simulink library "sm_trackV_lib_chain_underc_i2u0l4"  (R2026a)
settings: Solver=VariableStepAuto
undefined symbols (not defined in the file): Excv, P1, P2, P3, P4, Right
libraries: sm_trackV_lib_chain_underc_elem x9, sm_lib x8, nesl_utility x7, fl_lib x2, sm_trackV_lib_frame_i2u0l4 x1
Description:
  | Copyright 2023-2026 The MathWorks, Inc.
settings Model: Creator=smiller  LastModifiedBy=smiller

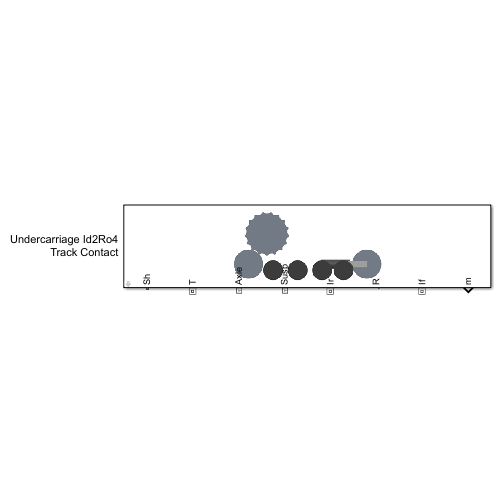
[thumbnail: Simulink's stored preview of the top-level diagram]
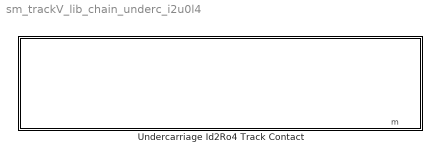
== system sm_trackV_lib_chain_underc_i2u0l4 ==
  Undercarriage Id2Ro4 Track Contact : Subsystem  mask(Undercarriage for Integration with Track Model){popup_leftOrRight=Right, sprk_xc=Excv.Sprocket.sprocket_xc, sprk_len=Excv.Sprocket.sprk_width, sprk_rho=Excv.Sprocket.density, sprk_clr=Excv.Sprocket.clr, sprk_opc=Excv.Sprocket.opc, sprk_contact_geo_ptcld=Excv.Sprocket.teeth_contact.ptcld.pts, sprk_contact_geo_rad=Excv.Sprocket.teeth_contact.ptcld.rad, sprk_contact_geo_clr=Excv.Sprocket.teeth_contact.ptcld.clr, sprk_contact_geo_opc=Excv.Sprocket.teeth_contact.ptcld.opc, idlerR_rad=Excv.IdlerR.rad, idlerF_rad=Excv.IdlerF.rad, idlerR_len=Excv.IdlerR.len, idlerF_len=Excv.IdlerF.len, idlerR_rho=Excv.IdlerR.rho, idlerF_rho=Excv.IdlerF.rho, idlerR_clr=Excv.IdlerR.clr, idlerF_clr=Excv.IdlerF.clr, idlerR_opc=Excv.IdlerR.opc, idlerF_opc=Excv.IdlerF.opc, idlerR_contgeo_clr=Excv.IdlerR.chain_contact.clr, idlerF_contgeo_clr=Excv.IdlerF.chain_contact.clr, idlerR_contgeo_opc=Excv.IdlerR.chain_contact.opc, idlerF_contgeo_opc=Excv.IdlerF.chain_contact.opc, roller_lower_rad=Excv.Roller.Lower.rad, roller_lower_len=Excv.Roller.Lower.len, roller_lower_rho=Excv.Roller.Lower.rho, roller_lower_clr=Excv.Roller.Lower.clr, roller_lower_opc=Excv.Roller.Lower.opc, roller_lower_contgeo_clr=[1.0 0.0 0.0], roller_lower_contgeo_opc=1, tensioner_cyl_len=Excv.IdlerF.Tensioner.cyl.len, tensioner_cyl_rad=Excv.IdlerF.Tensioner.cyl.rad, tensioner_cyl_rho=Excv.IdlerF.Tensioner.cyl.rho, tensioner_cyl_clr=Excv.IdlerF.Tensioner.cyl.clr, tensioner_cyl_opc=Excv.IdlerF.Tensioner.cyl.opc, tensioner_pist_len=Excv.IdlerF.Tensioner.piston.len, tensioner_pist_rad=Excv.IdlerF.Tensioner.piston.rad, tensioner_pist_rho=Excv.IdlerF.Tensioner.piston.rho, tensioner_pist_clr=Excv.IdlerF.Tensioner.piston.clr, tensioner_pist_opc=Excv.IdlerF.Tensioner.piston.opc, tensioner_br_len=Excv.IdlerF.Tensioner.bracket.len, tensioner_br_width=Excv.IdlerF.Tensioner.bracket.wid, tensioner_br_height=Excv.IdlerF.Tensioner.bracket.height, tensioner_br_thk=Excv.IdlerF.Tensioner.bracket.thk, tensioner_br_rho=Excv.IdlerF.Tensioner.bracket.rho, tensioner_br_clr=Excv.IdlerF.Tensioner.bracket.clr, tensioner_br_opc=Excv.IdlerF.Tensioner.bracket.opc, tensioner_eqpos=Excv.IdlerF.Tensioner.xeq, tensioner_x0=Excv.IdlerF.Tensioner.x0, tensioner_k=Excv.IdlerF.Tensioner.K, tensioner_b=Excv.IdlerF.Tensioner.B, roller_lower_x=Excv.Frame.Sprk2LowerX, idlerF_x=Excv.Frame.IdlerAssyX, idlerR_x=Excv.Frame.Sprk2IdlerRX, axle_x=Excv.Frame.AxleX, roller_lower_y=Excv.Frame.Sprk2LowerY, idlerF_y=Excv.Frame.Sprk2IdlerFY, idlerR_y=Excv.Frame.Sprk2IdlerFY, axle_y=Excv.Frame.AxleY, frame_cg_offset=Excv.Frame.CGOffset, frame_mass=Excv.Frame.Mass, frame_moi=Excv.Frame.MOI, frame_poi=Excv.Frame.POI, frame_susp_offset=Excv.Frame.SuspOffset, popup_sense_roller=Actuator Torque}
      mask prompts: popup_leftOrRight "Left or Right"; sprk_xc "Extrusion Data [x y] (m)"; sprk_len "Length (m)"; sprk_rho "Density (kg/m^3)"; sprk_clr "Color [R G B] (0-1)"; sprk_opc "Opacity (0-1)"; sprk_contact_geo_ptcld "Point Cloud Data [x y z] (m)"; sprk_contact_geo_rad "Radius (m)"; sprk_contact_geo_clr "Color [R G B] (0-1)"; sprk_contact_geo_opc "Opacity (0-1)"; roller_lower_rad "Radius (m)"; roller_lower_len "Length (m)"; roller_lower_rho "Density (kg/m^3)"; roller_lower_clr "Color [R G B] (0-1)"; roller_lower_opc "Opacity (0-1)"; roller_lower_contgeo_clr "Color [R G B] (0-1)"; roller_lower_contgeo_opc "Opacity (0-1)"; tensioner_cyl_len "Length (m)"; tensioner_cyl_rad "Radius (m)"; tensioner_cyl_rho "Density (kg/m^3)"; tensioner_cyl_clr "Color [R G B] (0-1)"; tensioner_cyl_opc "Opacity (0-1)"; tensioner_pist_len "Piston Length (m)"; tensioner_pist_rad "Radius (m)"; tensioner_pist_rho "Density (kg/m^3)"; tensioner_pist_clr "Color [R G B] (0-1)"; tensioner_pist_opc "Opacity (0.1)"; tensioner_br_len "Length (m)"; tensioner_br_width "Width (m)"; tensioner_br_height "Height (m)"; tensioner_br_thk "Bracket Thickness (m)"; tensioner_br_rho "Density (kg/m^3)"; tensioner_br_clr "Color [R G B] (0-1)"; tensioner_br_opc "Opacity (0.1)"; tensioner_eqpos "Equilibrium Position (m)"; tensioner_x0 "Assembly Position (m)"; tensioner_k "Stiffness Coefficient (N/m)"; tensioner_b "Damping Coefficient (N/(m/s))"; roller_lower_x "Lower Rollers (vector) (m)"; idlerF_x "Idler Wheel Front (m)"; idlerR_x "Idler Wheel Rear (m)"; axle_x "Axle (m)"; roller_lower_y "Lower Rollers (m)"; idlerF_y "Idler Front (m)"; idlerR_y "Idler Rear (m)"; axle_y "Axle (m)"; frame_cg_offset "CG Offset from Sprocket [x y z] (m)"; frame_mass "Mass (kg)"; frame_moi "Moments of Inertia [Ixx Iyy Izz] (kg*m^2)"; frame_poi "Products of Inertia [Ixx Iyy Izz] (kg*m^2)"; frame_susp_offset "Suspension Offset from Sprocket [x y z] (m)"; popup_sense_roller "Roller"
      mask help: Models sprocket, rollers, and idler with tensioner. Components have contact geometry for integration with a segmented track model. The sprocket has a 1D rotational mechanical interface to the drivetrain.
      mask init:
      | bh = gcb;
      | set_param([bh '/Rollers'],'popup_sense_roller',get_param(bh,'popup_sense_roller'));
      mask TypeOptions popup_leftOrRight: Frame/popup_leftOrRight
      mask TypeOptions sprk_xc: Rollers/sprk_xc
      mask TypeOptions sprk_len: Rollers/sprk_len
      mask TypeOptions sprk_rho: Rollers/sprk_rho
      mask TypeOptions sprk_clr: Rollers/sprk_clr
      mask TypeOptions sprk_opc: Rollers/sprk_opc
      mask TypeOptions sprk_contact_geo_ptcld: Rollers/sprk_contact_geo_ptcld
      mask TypeOptions sprk_contact_geo_rad: Rollers/sprk_contact_geo_rad
      mask TypeOptions sprk_contact_geo_clr: Rollers/sprk_contact_geo_clr
      mask TypeOptions sprk_contact_geo_opc: Rollers/sprk_contact_geo_opc
      mask TypeOptions idlerR_rad: Rollers/idlerR_rad
      mask TypeOptions idlerF_rad: Rollers/idlerF_rad
      mask TypeOptions idlerR_len: Rollers/idlerR_len
      mask TypeOptions idlerF_len: Rollers/idlerF_len
      mask TypeOptions idlerR_rho: Rollers/idlerR_rho
      mask TypeOptions idlerF_rho: Rollers/idlerF_rho
      mask TypeOptions idlerR_clr: Rollers/idlerR_clr
      mask TypeOptions idlerF_clr: Rollers/idlerF_clr
      mask TypeOptions idlerR_opc: Rollers/idlerR_opc
      mask TypeOptions idlerF_opc: Rollers/idlerF_opc
      mask TypeOptions idlerR_contgeo_clr: Rollers/idlerR_contgeo_clr
      mask TypeOptions idlerF_contgeo_clr: Rollers/idlerF_contgeo_clr
      mask TypeOptions idlerR_contgeo_opc: Rollers/idlerR_contgeo_opc
      mask TypeOptions idlerF_contgeo_opc: Rollers/idlerF_contgeo_opc
      mask TypeOptions roller_lower_rad: Rollers/roller_lower_rad
      mask TypeOptions roller_lower_len: Rollers/roller_lower_len
      mask TypeOptions roller_lower_rho: Rollers/roller_lower_rho
      mask TypeOptions roller_lower_clr: Rollers/roller_lower_clr
      mask TypeOptions roller_lower_opc: Rollers/roller_lower_opc
      mask TypeOptions roller_lower_contgeo_clr: Rollers/roller_lower_contgeo_clr
      mask TypeOptions roller_lower_contgeo_opc: Rollers/roller_lower_contgeo_opc
      mask TypeOptions tensioner_cyl_len: Rollers/tensioner_cyl_len
      mask TypeOptions tensioner_cyl_rad: Rollers/tensioner_cyl_rad
      mask TypeOptions tensioner_cyl_rho: Rollers/tensioner_cyl_rho
      mask TypeOptions tensioner_cyl_clr: Rollers/tensioner_cyl_clr
      mask TypeOptions tensioner_cyl_opc: Rollers/tensioner_cyl_opc
      mask TypeOptions tensioner_pist_len: Rollers/pist_len
      mask TypeOptions tensioner_pist_rad: Rollers/tensioner_pist_rad
      mask TypeOptions tensioner_pist_rho: Rollers/tensioner_pist_rho
      mask TypeOptions tensioner_pist_clr: Rollers/tensioner_pist_clr
      mask TypeOptions tensioner_pist_opc: Rollers/tensioner_pist_opc
      mask TypeOptions tensioner_br_len: Rollers/brk_len
      mask TypeOptions tensioner_br_width: Rollers/tensioner_br_width
      mask TypeOptions tensioner_br_height: Rollers/tensioner_br_height
      mask TypeOptions tensioner_br_thk: Rollers/brk_thk
      mask TypeOptions tensioner_br_rho: Rollers/tensioner_br_rho
      mask TypeOptions tensioner_br_clr: Rollers/tensioner_br_clr
      mask TypeOptions tensioner_br_opc: Rollers/tensioner_br_opc
      mask TypeOptions tensioner_eqpos: Rollers/tensioner_eqpos
      mask TypeOptions tensioner_x0: Rollers/tensioner_x0
      mask TypeOptions tensioner_k: Rollers/tensioner_k
      mask TypeOptions tensioner_b: Rollers/tensioner_b
      mask TypeOptions roller_lower_x: Frame/roller_lower_x
      mask TypeOptions idlerF_x: Frame/idlerF_x
      mask TypeOptions idlerR_x: Frame/idlerR_x
      mask TypeOptions axle_x: Frame/axle_x
      mask TypeOptions roller_lower_y: Frame/roller_lower_y
      mask TypeOptions idlerF_y: Frame/idlerF_y
      mask TypeOptions idlerR_y: Frame/idlerR_y
      mask TypeOptions axle_y: Frame/axle_y
      mask TypeOptions frame_cg_offset: Frame/frame_cg_offset
      mask TypeOptions frame_mass: Frame/frame_mass
      mask TypeOptions frame_moi: Frame/frame_moi
      mask TypeOptions frame_poi: Frame/frame_poi
      mask TypeOptions frame_susp_offset: Frame/frame_susp_offset
      mask TypeOptions popup_sense_roller: Constraint Force | Actuator Torque
      mask DialogControl cont_sprocket Prompt: Sprocket
      mask DialogControl cont_sprocket_solid Prompt: Solid
      mask DialogControl cont_sprocket_contact_geo Prompt: Contact Geometry
      mask DialogControl cont_idler Prompt: Idler
      mask DialogControl cont_idler_solid Prompt: Solid
      mask DialogControl text_rear Prompt: Rear
      mask DialogControl text_front Prompt: Front
      mask DialogControl text_rad Prompt: Radius (m)
      mask DialogControl text_len Prompt: Length (m)
      mask DialogControl text_rho Prompt: Density (kg/m^3)
      mask DialogControl text_clr Prompt: Color [R G B] (0-1)
      mask DialogControl text_opc Prompt: Opacity (0-1)
      mask DialogControl cont_idler_contact_geo Prompt: Contact Geometry
      mask DialogControl text_contgeo_clr Prompt: Color [R G B] (0-1)
      mask DialogControl text_contgeo_opc Prompt: Opacity (0-1)
      mask DialogControl cont_rollers Prompt: Rollers
      mask DialogControl cont_rollers_lower Prompt: Lower
      mask DialogControl cont_rollers_lower_contact_geo Prompt: Contact Geometry
      mask DialogControl cont_tensioner Prompt: Tensioner
      mask DialogControl cont_tensioner_cyl Prompt: Cylinder
      mask DialogControl cont_tensioner_pist Prompt: Piston
      mask DialogControl cont_tensioner_brkt Prompt: Bracket
      mask DialogControl cont_tensioner_assembly Prompt: Assembly
      mask DialogControl cont_frame Prompt: Frame
      mask DialogControl cont_offset_x Prompt: Longitudinal Offsets from Sprocket
      mask DialogControl cont_offset_y Prompt: Vertical Offsets
      mask DialogControl cont_mass Prompt: Mass and Inertia
      mask DialogControl cont_susp Prompt: Suspension Offsets
      mask DialogControl cont_sensing Prompt: Sensing
      mask Display: image('sm_chain_underc_i2u0l4_IMAGE.png');

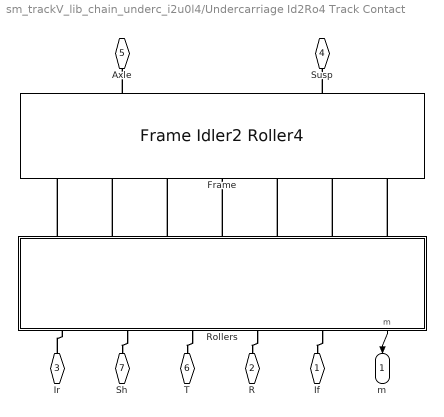
== system sm_trackV_lib_chain_underc_i2u0l4/Undercarriage Id2Ro4 Track Contact ==
  Frame : sm_trackV_lib_frame_i2u0l4/Frame Idler2 Roller4  popup_leftOrRight=Right  roller_lower_x=roller_lower_x  idlerF_x=idlerF_x  idlerR_x=idlerR_x  axle_x=axle_x  roller_lower_y=roller_lower_y  idlerF_y=idlerF_y  idlerR_y=idlerR_y  axle_y=axle_y  frame_cg_offset=frame_cg_offset  frame_mass=frame_mass  frame_moi=frame_moi  frame_poi=frame_poi  frame_susp_offset=frame_susp_offset
  Rollers : Subsystem  mask(Rollers for Integration with Track Model){sprk_xc=sprk_xc, sprk_len=sprk_len, sprk_rho=sprk_rho, sprk_clr=sprk_clr, sprk_opc=sprk_opc, sprk_contact_geo_ptcld=sprk_contact_geo_ptcld, sprk_contact_geo_rad=sprk_contact_geo_rad, sprk_contact_geo_clr=sprk_contact_geo_clr, sprk_contact_geo_opc=sprk_contact_geo_opc, idlerR_rad=idlerR_rad, idlerF_rad=idlerF_rad, idlerR_len=idlerR_len, idlerF_len=idlerF_len, idlerR_rho=idlerR_rho, idlerF_rho=idlerF_rho, idlerR_clr=idlerR_clr, idlerF_clr=idlerF_clr, idlerR_opc=idlerR_opc, idlerF_opc=idlerF_opc, idlerR_contgeo_clr=idlerR_contgeo_clr, idlerF_contgeo_clr=idlerF_contgeo_clr, idlerR_contgeo_opc=idlerR_contgeo_opc, idlerF_contgeo_opc=idlerF_contgeo_opc, roller_lower_len=roller_lower_len, roller_lower_rad=roller_lower_rad, roller_lower_rho=roller_lower_rho, roller_lower_clr=roller_lower_clr, roller_lower_opc=roller_lower_opc, roller_lower_contgeo_clr=roller_lower_contgeo_clr, roller_lower_contgeo_opc=roller_lower_contgeo_opc, tensioner_cyl_rad=tensioner_cyl_rad, tensioner_cyl_len=tensioner_cyl_len, tensioner_cyl_rho=tensioner_cyl_rho, tensioner_cyl_clr=tensioner_cyl_clr, tensioner_cyl_opc=tensioner_cyl_opc, tensioner_pist_rad=tensioner_pist_rad, pist_len=tensioner_pist_len, tensioner_pist_rho=tensioner_pist_rho, tensioner_pist_clr=tensioner_pist_clr, tensioner_pist_opc=tensioner_pist_opc, brk_len=tensioner_br_len, tensioner_br_width=tensioner_br_width, tensioner_br_height=tensioner_br_height, brk_thk=tensioner_br_thk, tensioner_br_rho=tensioner_br_rho, tensioner_br_clr=tensioner_br_clr, tensioner_br_opc=tensioner_br_opc, tensioner_eqpos=tensioner_eqpos, tensioner_x0=tensioner_x0, tensioner_b=tensioner_b, tensioner_k=tensioner_k, popup_sense_roller=Actuator Torque}
      mask prompts: sprk_xc "Extrusion Data [x y] (m)"; sprk_len "Length (m)"; sprk_rho "Density (kg/m^3)"; sprk_clr "Color [R G B] (0-1)"; sprk_opc "Opacity (0-1)"; sprk_contact_geo_ptcld "Point Cloud Data [x y z] (m)"; sprk_contact_geo_rad "Radius (m)"; sprk_contact_geo_clr "Color [R G B] (0-1)"; sprk_contact_geo_opc "Opacity (0-1)"; roller_lower_len "Length (m)"; roller_lower_rad "Radius (m)"; roller_lower_rho "Density (kg/m^3)"; roller_lower_clr "Color [R G B] (0-1)"; roller_lower_opc "Opacity (0-1)"; roller_lower_contgeo_clr "Color [R G B] (0-1)"; roller_lower_contgeo_opc "Opacity (0-1)"; tensioner_cyl_rad "Radius (m)"; tensioner_cyl_len "Length (m)"; tensioner_cyl_rho "Density (kg/m^3)"; tensioner_cyl_clr "Color [R G B] (0-1)"; tensioner_cyl_opc "Opacity (0-1)"; tensioner_pist_rad "Radius (m)"; pist_len "Piston Length (m)"; tensioner_pist_rho "Density (kg/m^3)"; tensioner_pist_clr "Color [R G B] (0-1)"; tensioner_pist_opc "Opacity (0.1)"; brk_len "Bracket Length (m)"; tensioner_br_width "Width (m)"; tensioner_br_height "Height (m)"; brk_thk "Bracket Thickness (m)"; tensioner_br_rho "Density (kg/m^3)"; tensioner_br_clr "Color [R G B] (0-1)"; tensioner_br_opc "Opacity (0.1)"; tensioner_eqpos "Equilibrium Position (m)"; tensioner_x0 "Assembly Position (m)"; tensioner_b "Damping Coefficient (N/(m/s))"; tensioner_k "Stiffness Coefficient (N/m)"; popup_sense_roller "Roller"
      mask help: Models sprocket, rollers, and idler with tensioner. Components have contact geometry for integration with a segmented track model. The sprocket has a 1D rotational mechanical interface to the drivetrain.
      mask init:
      | % Sensing a constraint force can be computationally expensive
      | % Use popup to turn it off if quantity is not needed
      | bh = gcb;
      | if(strcmp(get_param(bh,'popup_sense_roller'),'Constraint Force'))
      |     SCF = 'on'; STF = 'off';
      |     connectedPort = "fc_out";
      |     senseConstraintTorque = "on";
      |     senseTorqueForce = "off";
      | else
      |     SCF = 'off'; STF = 'on';
      |     connectedPort = "t_out";
      |     senseConstraintTorque = "off";
      |     senseTorqueForce = "on";
      | end
      | f = Simulink.FindOptions('RegExp',true,'SearchDepth',1);
      | bh_rv = Simulink.findBlocks(bh,'Name','Revolute Lower #*',f);
      | bh_ps = Simulink.findBlocks(bh,'Name','PS-SL Lower #*',f);
      | [~, indrv] = sort(getfullname(bh_rv));
      | [~, indps] = sort(getfullname(bh_ps));
      | bh_rv = bh_rv(indrv);
      | bh_ps = bh_ps(indps);
      | 
      | bh_rvidf = get_param([bh '/Revolute Idler F'],'Handle');
      | bh_rvidr = get_param([bh '/Revolute Idler R'],'Handle');
      | 
      | bh_psidf = get_param([bh '/PS-SL IdlerF'],'Handle');
      | bh_psidr = get_param([bh '/PS-SL IdlerR'],'Handle');
      | 
      | bh_rv = [bh_rv; bh_rvidr; bh_rvidf];
      | bh_ps = [bh_ps; bh_psidr; bh_psidf];
      | 
      | for i = 1:length(bh_rv)
      |     port_rv = get_param(bh_rv(i),'PortHandles');
      |     port_ps = get_param(bh_ps(i),'PortHandles');
      |     line_rv = get_param(bh_rv(i),'LineHandles');
      |     delete_line(line_rv.RConn(2))
      |     set_param(bh_rv(i),'SenseConstraintForce',SCF,'SenseTorqueForce',STF);
      |     %port_rv = get_param(bh_rv(1),'PortHandles')
      |     %add_line(bh,port_rv.RConn(2),port_ps.LConn,'autorouting','on');
      |     simscape.addConnection(bh_rv(i), connectedPort, bh_ps(i),'input');
      | end
      mask TypeOptions sprk_xc: Sprocket/sprk_xc
      mask TypeOptions sprk_len: Sprocket/sprk_len
      mask TypeOptions sprk_rho: Sprocket/sprk_rho
      mask TypeOptions sprk_clr: Sprocket/sprk_clr
      mask TypeOptions sprk_opc: Sprocket/sprk_opc
      mask TypeOptions sprk_contact_geo_ptcld: Sprocket/sprk_contact_geo_ptcld
      mask TypeOptions sprk_contact_geo_rad: Sprocket/sprk_contact_geo_rad
      mask TypeOptions sprk_contact_geo_clr: Sprocket/sprk_contact_geo_clr
      mask TypeOptions sprk_contact_geo_opc: Sprocket/sprk_contact_geo_opc
      mask TypeOptions idlerR_rad: IdlerR/idler_rad
      mask TypeOptions idlerF_rad: IdlerF/idler_rad
      mask TypeOptions idlerR_len: IdlerR/idler_len
      mask TypeOptions idlerF_len: IdlerF/idler_len
      mask TypeOptions idlerR_rho: IdlerR/idler_rho
      mask TypeOptions idlerF_rho: IdlerF/idler_rho
      mask TypeOptions idlerR_clr: IdlerR/idler_clr
      mask TypeOptions idlerF_clr: IdlerF/idler_clr
      mask TypeOptions idlerR_opc: IdlerR/idler_opc
      mask TypeOptions idlerF_opc: IdlerF/idler_opc
      mask TypeOptions idlerR_contgeo_clr: IdlerR/idler_contgeo_clr
      mask TypeOptions idlerF_contgeo_clr: IdlerF/idler_contgeo_clr
      mask TypeOptions idlerR_contgeo_opc: IdlerR/idler_contgeo_opc
      mask TypeOptions idlerF_contgeo_opc: IdlerF/idler_contgeo_opc
      mask TypeOptions roller_lower_len:
      | Roller
      | Lower 1/roller_lower_len | Roller
      | Lower 2/roller_lower_len | Roller
      | Lower 3/roller_lower_len | Roller
      | Lower 4/roller_lower_len
      mask TypeOptions roller_lower_rad:
      | Roller
      | Lower 1/roller_lower_rad | Roller
      | Lower 2/roller_lower_rad | Roller
      | Lower 3/roller_lower_rad | Roller
      | Lower 4/roller_lower_rad
      mask TypeOptions roller_lower_rho:
      | Roller
      | Lower 1/roller_lower_rho | Roller
      | Lower 2/roller_lower_rho | Roller
      | Lower 3/roller_lower_rho | Roller
      | Lower 4/roller_lower_rho
      mask TypeOptions roller_lower_clr:
      | Roller
      | Lower 1/roller_lower_clr | Roller
      | Lower 2/roller_lower_clr | Roller
      | Lower 3/roller_lower_clr | Roller
      | Lower 4/roller_lower_clr
      mask TypeOptions roller_lower_opc:
      | Roller
      | Lower 1/roller_lower_opc | Roller
      | Lower 2/roller_lower_opc | Roller
      | Lower 3/roller_lower_opc | Roller
      | Lower 4/roller_lower_opc
      mask TypeOptions roller_lower_contgeo_clr:
      | Roller
      | Lower 1/roller_lower_contgeo_clr | Roller
      | Lower 2/roller_lower_contgeo_clr | Roller
      | Lower 3/roller_lower_contgeo_clr | Roller
      | Lower 4/roller_lower_contgeo_clr
      mask TypeOptions roller_lower_contgeo_opc:
      | Roller
      | Lower 1/roller_lower_contgeo_opc | Roller
      | Lower 2/roller_lower_contgeo_opc | Roller
      | Lower 3/roller_lower_contgeo_opc | Roller
      | Lower 4/roller_lower_contgeo_opc
      mask TypeOptions tensioner_cyl_rad:
      | Tensioner
      | Cylinder/cyl_rad
      mask TypeOptions tensioner_cyl_len:
      | Tensioner
      | Cylinder/cyl_len
      mask TypeOptions tensioner_cyl_rho:
      | Tensioner
      | Cylinder/cyl_rho
      mask TypeOptions tensioner_cyl_clr:
      | Tensioner
      | Cylinder/cyl_clr
      mask TypeOptions tensioner_cyl_opc:
      | Tensioner
      | Cylinder/cyl_opc
      mask TypeOptions tensioner_pist_rad:
      | Tensioner
      | Piston/pist_rad
      mask TypeOptions pist_len:
      | Tensioner
      | Cylinder/pist_len | Tensioner
      | Piston/pist_len
      mask TypeOptions tensioner_pist_rho:
      | Tensioner
      | Piston/pist_rho
      mask TypeOptions tensioner_pist_clr:
      | Tensioner
      | Piston/pist_clr
      mask TypeOptions tensioner_pist_opc:
      | Tensioner
      | Piston/pist_opc
      mask TypeOptions brk_len:
      | Tensioner
      | Cylinder/brk_len | Tensioner
      | Piston/br_length
      mask TypeOptions tensioner_br_width:
      | Tensioner
      | Piston/br_width
      mask TypeOptions tensioner_br_height:
      | Tensioner
      | Piston/br_height
      mask TypeOptions brk_thk:
      | Tensioner
      | Cylinder/brk_thk | Tensioner
      | Piston/br_thk
      mask TypeOptions tensioner_br_rho:
      | Tensioner
      | Piston/br_rho
      mask TypeOptions tensioner_br_clr:
      | Tensioner
      | Piston/br_clr
      mask TypeOptions tensioner_br_opc:
      | Tensioner
      | Piston/br_opc
      mask TypeOptions tensioner_eqpos:
      | Prismatic
      | Tensioner/EquilibriumPosition
      mask TypeOptions tensioner_x0:
      | Prismatic
      | Tensioner/PositionTargetValue
      mask TypeOptions tensioner_b:
      | Prismatic
      | Tensioner/DampingCoefficient
      mask TypeOptions tensioner_k:
      | Prismatic
      | Tensioner/SpringStiffness
      mask TypeOptions popup_sense_roller: Constraint Force | Actuator Torque
      mask DialogControl cont_sprk Prompt: Sprocket
      mask DialogControl cont_sprk_solid Prompt: Solid
      mask DialogControl cont_sprk_contact_geo Prompt: Contact Geometry
      mask DialogControl cont_idler Prompt: Idler
      mask DialogControl cont_idler_solid Prompt: Solid
      mask DialogControl text_idler_rear Prompt: Rear
      mask DialogControl text_idler_front Prompt: Front
      mask DialogControl text_radius Prompt: Radius (m)
      mask DialogControl text_len Prompt: Length(m)
      mask DialogControl text_rho Prompt: Density (kg/m^3)
      mask DialogControl text_clr Prompt: Color [R G B] (0-1)
      mask DialogControl text_opc Prompt: Opacity (0-1)
      mask DialogControl cont_idler_contact_geo Prompt: Contact Geometry
      mask DialogControl Control10 Prompt: Color [R G B] (0-1)
      mask DialogControl text_contgeo_opc Prompt: Opacity (0-1)
      mask DialogControl cont_rollers Prompt: Rollers
      mask DialogControl cont_lower Prompt: Lower
      mask DialogControl cont_lower_contact_geo Prompt: Contact Geometry
      mask DialogControl cont_tensioner Prompt: Tensioner
      mask DialogControl cont_tensioner_cyl Prompt: Cylinder
      mask DialogControl cont_tensioner_pist Prompt: Piston
      mask DialogControl cont_tensioner_brkt Prompt: Bracket
      mask DialogControl cont_tensioner_assy Prompt: Assembly
      mask DialogControl Container20 Prompt: Sensing
      mask Display: image('sm_chain_underc_i2u0l4_IMAGE.png');
  If : PMIOPort  Side=Right
  R : PMIOPort  Port=2  Side=Right
  Ir : PMIOPort  Port=3  Side=Right
  Susp : PMIOPort  Port=4  Side=Right
  Axle : PMIOPort  Port=5  Side=Right
  T : PMIOPort  Port=6  Side=Right
  Sh : PMIOPort  Port=7  Side=Right
  m : Outport
  wires:
  Rollers/1(m) -> m/1
  connections:
  Ir/RConn1 -- Rollers/RConn5
  Rollers/LConn1 -- Frame/RConn1
  Rollers/LConn2 -- Frame/RConn2
  Rollers/LConn3 -- Frame/RConn3
  Rollers/LConn4 -- Frame/RConn4
  Rollers/LConn5 -- Frame/RConn5
  Rollers/LConn6 -- Frame/RConn6
  Rollers/LConn7 -- Frame/RConn7
  Frame/LConn1 -- Susp/RConn1
  Rollers/RConn2 -- R/RConn1
  Frame/LConn2 -- Axle/RConn1
  Rollers/RConn1 -- If/RConn1
  Rollers/RConn3 -- T/RConn1
  Rollers/RConn4 -- Sh/RConn1

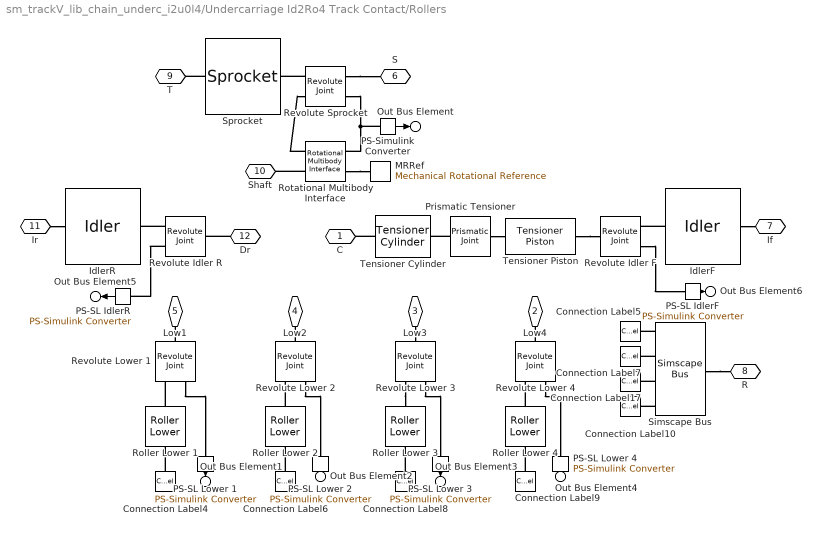
== system sm_trackV_lib_chain_underc_i2u0l4/Undercarriage Id2Ro4 Track Contact/Rollers ==
  Connection Label10 : ConnectionLabel  Label=L4
  Connection Label17 : ConnectionLabel  Label=L3
  Connection Label4 : ConnectionLabel  Label=L1
  Connection Label5 : ConnectionLabel  Label=L1
  Connection Label6 : ConnectionLabel  Label=L2
  Connection Label7 : ConnectionLabel  Label=L2
  Connection Label8 : ConnectionLabel  Label=L3
  Connection Label9 : ConnectionLabel  Label=L4
  IdlerF : sm_trackV_lib_chain_underc_elem/Idler  idler_rad=idlerF_rad  idler_len=idlerF_len  idler_rho=idlerF_rho  idler_clr=idlerF_clr  idler_opc=idlerF_opc  idler_contgeo_clr=idlerF_contgeo_clr  idler_contgeo_opc=idlerF_contgeo_opc
  IdlerR : sm_trackV_lib_chain_underc_elem/Idler  idler_rad=idlerR_rad  idler_len=idlerR_len  idler_rho=idlerR_rho  idler_clr=idlerR_clr  idler_opc=idlerR_opc  idler_contgeo_clr=idlerR_contgeo_clr  idler_contgeo_opc=idlerR_contgeo_opc
  MRRef : fl_lib/Mechanical/Rotational Elements/Mechanical Rotational Reference
  PS-SL IdlerF : nesl_utility/PS-Simulink Converter  PhysicalDomain=network_engine_domain  SubClassName=ps_output  LeftPortType=input  RightPortType=output  PseudoPeriodic=off  Frequencies=[]  VectorFormat=inherit  Unit=inherit  AffineConversion=off
  PS-SL IdlerR : nesl_utility/PS-Simulink Converter  PhysicalDomain=network_engine_domain  SubClassName=ps_output  LeftPortType=input  RightPortType=output  PseudoPeriodic=off  Frequencies=[]  VectorFormat=inherit  Unit=inherit  AffineConversion=off
  PS-SL Lower {1..4} (4 alike) : nesl_utility/PS-Simulink Converter  PhysicalDomain=network_engine_domain  SubClassName=ps_output  LeftPortType=input  RightPortType=output  PseudoPeriodic=off  Frequencies=[]  VectorFormat=inherit  Unit=inherit  AffineConversion=off
  PS-Simulink Converter : nesl_utility/PS-Simulink Converter  PhysicalDomain=network_engine_domain  SubClassName=ps_output  LeftPortType=input  RightPortType=output  PseudoPeriodic=off  Frequencies=[]  VectorFormat=inherit  Unit=inherit  AffineConversion=off
  Prismatic Tensioner : sm_lib/Joints/Prismatic Joint  JointMode=Normal  CompositeWrenchDir=FollowerOnBase  CompositeWrenchFrame=BaseFrame  SenseConstraintForce=off  SenseConstraintTorque=off  SenseTotalForce=off  SenseTotalTorque=off  PositionTargetSpecify=on  PositionTargetPriority=High  PositionTargetValue=tensioner_x0  PositionTargetValueUnits=m  VelocityTargetSpecify=off  VelocityTargetPriority=High  VelocityTargetValue=0  VelocityTargetValueUnits=m/s  EquilibriumPosition=tensioner_eqpos  EquilibriumPositionUnits=m  SpringStiffness=tensioner_k  SpringStiffnessUnits=N/m  DampingCoefficient=tensioner_b  DampingCoefficientUnits=N/(m/s)  LowerLimitSpecify=off  LowerLimitBound=-1  LowerLimitBoundUnits=m  LowerLimitStiffness=1e6  LowerLimitStiffnessUnits=N/m  LowerLimitDamping=1e3  LowerLimitDampingUnits=N/(m/s)  LowerLimitTransitionRegionWidth=1e-4  LowerLimitTransitionRegionWidthUnits=m  UpperLimitSpecify=off  UpperLimitBound=1  UpperLimitBoundUnits=m  UpperLimitStiffness=1e6  UpperLimitStiffnessUnits=N/m  UpperLimitDamping=1e3  UpperLimitDampingUnits=N/(m/s)  UpperLimitTransitionRegionWidth=1e-4  UpperLimitTransitionRegionWidthUnits=m  TorqueActuationMode=NoTorque  MotionActuationMode=ComputedMotion  SensePosition=off  SenseVelocity=off  SenseAcceleration=off  SenseTorqueForce=off  SenseLowerLimitTorqueForce=off  SenseUpperLimitTorqueForce=off
  Revolute Idler F : sm_lib/Joints/Revolute Joint  JointMode=Normal  CompositeWrenchDir=FollowerOnBase  CompositeWrenchFrame=BaseFrame  SenseConstraintForce=off  SenseConstraintTorque=off  SenseTotalForce=off  SenseTotalTorque=off  PositionTargetSpecify=off  PositionTargetPriority=Low  PositionTargetValue=0  PositionTargetValueUnits=deg  VelocityTargetSpecify=off  VelocityTargetPriority=High  VelocityTargetValue=0  VelocityTargetValueUnits=deg/s  EquilibriumPosition=0  EquilibriumPositionUnits=rad  SpringStiffness=0  SpringStiffnessUnits=N*m/rad  DampingCoefficient=0  DampingCoefficientUnits=N*m/(rad/s)  LowerLimitSpecify=off  LowerLimitBound=-90  LowerLimitBoundUnits=deg  LowerLimitStiffness=1e4  LowerLimitStiffnessUnits=N*m/deg  LowerLimitDamping=10  LowerLimitDampingUnits=N*m/(deg/s)  LowerLimitTransitionRegionWidth=0.1  LowerLimitTransitionRegionWidthUnits=deg  UpperLimitSpecify=off  UpperLimitBound=90  UpperLimitBoundUnits=deg  UpperLimitStiffness=1e4  UpperLimitStiffnessUnits=N*m/deg  UpperLimitDamping=10  UpperLimitDampingUnits=N*m/(deg/s)  UpperLimitTransitionRegionWidth=0.1  UpperLimitTransitionRegionWidthUnits=deg  TorqueActuationMode=NoTorque  MotionActuationMode=ComputedMotion  SensePosition=off  SenseVelocity=off  SenseAcceleration=off  SenseTorqueForce=on  SenseLowerLimitTorqueForce=off  SenseUpperLimitTorqueForce=off
  Revolute Idler R : sm_lib/Joints/Revolute Joint  JointMode=Normal  CompositeWrenchDir=FollowerOnBase  CompositeWrenchFrame=BaseFrame  SenseConstraintForce=off  SenseConstraintTorque=off  SenseTotalForce=off  SenseTotalTorque=off  PositionTargetSpecify=off  PositionTargetPriority=Low  PositionTargetValue=0  PositionTargetValueUnits=deg  VelocityTargetSpecify=off  VelocityTargetPriority=High  VelocityTargetValue=0  VelocityTargetValueUnits=deg/s  EquilibriumPosition=0  EquilibriumPositionUnits=rad  SpringStiffness=0  SpringStiffnessUnits=N*m/rad  DampingCoefficient=0  DampingCoefficientUnits=N*m/(rad/s)  LowerLimitSpecify=off  LowerLimitBound=-90  LowerLimitBoundUnits=deg  LowerLimitStiffness=1e4  LowerLimitStiffnessUnits=N*m/deg  LowerLimitDamping=10  LowerLimitDampingUnits=N*m/(deg/s)  LowerLimitTransitionRegionWidth=0.1  LowerLimitTransitionRegionWidthUnits=deg  UpperLimitSpecify=off  UpperLimitBound=90  UpperLimitBoundUnits=deg  UpperLimitStiffness=1e4  UpperLimitStiffnessUnits=N*m/deg  UpperLimitDamping=10  UpperLimitDampingUnits=N*m/(deg/s)  UpperLimitTransitionRegionWidth=0.1  UpperLimitTransitionRegionWidthUnits=deg  TorqueActuationMode=NoTorque  MotionActuationMode=ComputedMotion  SensePosition=off  SenseVelocity=off  SenseAcceleration=off  SenseTorqueForce=on  SenseLowerLimitTorqueForce=off  SenseUpperLimitTorqueForce=off
  Revolute Lower {1..4} (4 alike) : sm_lib/Joints/Revolute Joint  JointMode=Normal  CompositeWrenchDir=FollowerOnBase  CompositeWrenchFrame=BaseFrame  SenseConstraintForce=off  SenseConstraintTorque=off  SenseTotalForce=off  SenseTotalTorque=off  PositionTargetSpecify=off  PositionTargetPriority=Low  PositionTargetValue=0  PositionTargetValueUnits=deg  VelocityTargetSpecify=off  VelocityTargetPriority=High  VelocityTargetValue=0  VelocityTargetValueUnits=deg/s  EquilibriumPosition=0  EquilibriumPositionUnits=rad  SpringStiffness=0  SpringStiffnessUnits=N*m/rad  DampingCoefficient=0  DampingCoefficientUnits=N*m/(rad/s)  LowerLimitSpecify=off  LowerLimitBound=-90  LowerLimitBoundUnits=deg  LowerLimitStiffness=1e4  LowerLimitStiffnessUnits=N*m/deg  LowerLimitDamping=10  LowerLimitDampingUnits=N*m/(deg/s)  LowerLimitTransitionRegionWidth=0.1  LowerLimitTransitionRegionWidthUnits=deg  UpperLimitSpecify=off  UpperLimitBound=90  UpperLimitBoundUnits=deg  UpperLimitStiffness=1e4  UpperLimitStiffnessUnits=N*m/deg  UpperLimitDamping=10  UpperLimitDampingUnits=N*m/(deg/s)  UpperLimitTransitionRegionWidth=0.1  UpperLimitTransitionRegionWidthUnits=deg  TorqueActuationMode=NoTorque  MotionActuationMode=ComputedMotion  SensePosition=off  SenseVelocity=off  SenseAcceleration=off  SenseTorqueForce=on  SenseLowerLimitTorqueForce=off  SenseUpperLimitTorqueForce=off
  Revolute Sprocket : sm_lib/Joints/Revolute Joint  JointMode=Normal  CompositeWrenchDir=FollowerOnBase  CompositeWrenchFrame=BaseFrame  SenseConstraintForce=off  SenseConstraintTorque=off  SenseTotalForce=off  SenseTotalTorque=off  PositionTargetSpecify=off  PositionTargetPriority=Low  PositionTargetValue=0  PositionTargetValueUnits=deg  VelocityTargetSpecify=off  VelocityTargetPriority=High  VelocityTargetValue=0  VelocityTargetValueUnits=deg/s  EquilibriumPosition=0  EquilibriumPositionUnits=rad  SpringStiffness=0  SpringStiffnessUnits=N*m/rad  DampingCoefficient=0  DampingCoefficientUnits=N*m/(rad/s)  LowerLimitSpecify=off  LowerLimitBound=-90  LowerLimitBoundUnits=deg  LowerLimitStiffness=1e4  LowerLimitStiffnessUnits=N*m/deg  LowerLimitDamping=10  LowerLimitDampingUnits=N*m/(deg/s)  LowerLimitTransitionRegionWidth=0.1  LowerLimitTransitionRegionWidthUnits=deg  UpperLimitSpecify=off  UpperLimitBound=90  UpperLimitBoundUnits=deg  UpperLimitStiffness=1e4  UpperLimitStiffnessUnits=N*m/deg  UpperLimitDamping=10  UpperLimitDampingUnits=N*m/(deg/s)  UpperLimitTransitionRegionWidth=0.1  UpperLimitTransitionRegionWidthUnits=deg  TorqueActuationMode=InputTorque  MotionActuationMode=ComputedMotion  SensePosition=off  SenseVelocity=on  SenseAcceleration=off  SenseTorqueForce=off  SenseLowerLimitTorqueForce=off  SenseUpperLimitTorqueForce=off
  Roller Lower {1..4} (4 alike) : sm_trackV_lib_chain_underc_elem/Roller Lower  roller_lower_rad=roller_lower_rad  roller_lower_len=roller_lower_len  roller_lower_rho=roller_lower_rho  roller_lower_clr=roller_lower_clr  roller_lower_opc=roller_lower_opc  roller_lower_contgeo_clr=roller_lower_contgeo_clr  roller_lower_contgeo_opc=roller_lower_contgeo_opc
      settings: LibrarySourceBlock=sm_chain_drive_lib/Pulley_Bot
  Rotational Multibody Interface : fl_lib/Mechanical/Multibody Interfaces/Rotational Multibody Interface
  Simscape Bus : SimscapeBus  HierarchyStrings=P1;P2;P3;P4  ConnectionType=Bus: CBO_Roller4
  Sprocket : sm_trackV_lib_chain_underc_elem/Sprocket  sprk_xc=sprk_xc  sprk_len=sprk_len  sprk_rho=sprk_rho  sprk_clr=sprk_clr  sprk_opc=sprk_opc  sprk_contact_geo_ptcld=sprk_contact_geo_ptcld  sprk_contact_geo_rad=sprk_contact_geo_rad  sprk_contact_geo_clr=sprk_contact_geo_clr  sprk_contact_geo_opc=sprk_contact_geo_opc
  Tensioner Cylinder : sm_trackV_lib_chain_underc_elem/Tensioner Cylinder  cyl_rad=tensioner_cyl_rad  cyl_len=tensioner_cyl_len  cyl_rho=tensioner_cyl_rho  cyl_clr=tensioner_cyl_clr  cyl_opc=tensioner_cyl_opc  brk_len=brk_len  brk_thk=brk_thk  pist_len=pist_len
      settings: LibrarySourceBlock=sm_chain_drive_lib/Idler_Housing
  Tensioner Piston : sm_trackV_lib_chain_underc_elem/Tensioner Piston  pist_rad=tensioner_pist_rad  pist_len=pist_len  pist_rho=tensioner_pist_rho  pist_clr=tensioner_pist_clr  pist_opc=tensioner_pist_opc  br_height=tensioner_br_height  br_length=brk_len  br_width=tensioner_br_width  br_rho=tensioner_br_rho  br_thk=brk_thk  br_clr=tensioner_br_clr  br_opc=tensioner_br_opc
      settings: LibrarySourceBlock=sm_chain_drive_lib/ldler_Damper
  C : PMIOPort  Side=Left
  Low4 : PMIOPort  Port=2  Side=Left
  Low3 : PMIOPort  Port=3  Side=Left
  Low2 : PMIOPort  Port=4  Side=Left
  Low1 : PMIOPort  Port=5  Side=Left
  S : PMIOPort  Port=6  Side=Left
  If : PMIOPort  Port=7  Side=Right
  R : PMIOPort  Port=8  Side=Right
  T : PMIOPort  Port=9  Side=Right
  Shaft : PMIOPort  Port=10  Side=Right
  Ir : PMIOPort  Port=11  Side=Right
  Dr : PMIOPort  Port=12  Side=Left
  Out Bus Element : Outport  PortName=m  Element=tSprk
  Out Bus Element1 : Outport  PortName=m  Element=RL1
  Out Bus Element2 : Outport  PortName=m  Element=RL2
  Out Bus Element3 : Outport  PortName=m  Element=RL3
  Out Bus Element4 : Outport  PortName=m  Element=RL4
  Out Bus Element5 : Outport  PortName=m  Element=XIdlerR
  Out Bus Element6 : Outport  PortName=m  Element=XIdlerF
  wires:
  PS-SL Lower 4/1 -> Out Bus Element4/1
  PS-SL Lower 3/1 -> Out Bus Element3/1
  PS-SL Lower 2/1 -> Out Bus Element2/1
  PS-SL Lower 1/1 -> Out Bus Element1/1
  PS-Simulink Converter/1 -> Out Bus Element/1
  PS-SL IdlerR/1 -> Out Bus Element5/1
  PS-SL IdlerF/1 -> Out Bus Element6/1
  connections:
  Dr/RConn1 -- Revolute Idler R/LConn1
  Revolute Idler R/RConn1 -- IdlerR/LConn1
  Ir/RConn1 -- IdlerR/RConn1
  Rotational Multibody Interface/LConn2 -- MRRef/LConn1
  Rotational Multibody Interface/RConn2 -- Shaft/RConn1
  Rotational Multibody Interface/RConn1 -- Revolute Sprocket/RConn2
  PS-Simulink Converter/LConn1 -- Revolute Sprocket/LConn2 -- Rotational Multibody Interface/LConn1
  Roller Lower 4/LConn1 -- Revolute Lower 4/RConn1
  Roller Lower 1/LConn1 -- Revolute Lower 1/RConn1
  Low3/RConn1 -- Revolute Lower 3/LConn1
  Roller Lower 2/LConn1 -- Revolute Lower 2/RConn1
  Prismatic Tensioner/RConn1 -- Tensioner Piston/LConn1
  Tensioner Cylinder/LConn1 -- C/RConn1
  Simscape Bus/LConn1 -- Connection Label5/LConn1
  Simscape Bus/LConn2 -- Connection Label7/LConn1
  Simscape Bus/LConn3 -- Connection Label17/LConn1
  Simscape Bus/LConn4 -- Connection Label10/LConn1
  Revolute Lower 1/LConn1 -- Low1/RConn1
  Revolute Lower 3/RConn1 -- Roller Lower 3/LConn1
  Revolute Lower 4/LConn1 -- Low4/RConn1
  Connection Label4/LConn1 -- Roller Lower 1/RConn1
  Sprocket/RConn1 -- T/RConn1
  Tensioner Piston/RConn1 -- Revolute Idler F/LConn1
  Revolute Lower 2/LConn1 -- Low2/RConn1
  Prismatic Tensioner/LConn1 -- Tensioner Cylinder/RConn1
  Revolute Sprocket/RConn1 -- Sprocket/LConn1
  IdlerF/LConn1 -- Revolute Idler F/RConn1
  Simscape Bus/RConn1 -- R/RConn1
  Revolute Sprocket/LConn1 -- S/RConn1
  Connection Label8/LConn1 -- Roller Lower 3/RConn1
  Connection Label9/LConn1 -- Roller Lower 4/RConn1
  Connection Label6/LConn1 -- Roller Lower 2/RConn1
  IdlerF/RConn1 -- If/RConn1
  Revolute Lower 1/RConn2 -- PS-SL Lower 1/LConn1
  Revolute Lower 2/RConn2 -- PS-SL Lower 2/LConn1
  Revolute Lower 3/RConn2 -- PS-SL Lower 3/LConn1
  Revolute Lower 4/RConn2 -- PS-SL Lower 4/LConn1
  Revolute Idler R/RConn2 -- PS-SL IdlerR/LConn1
  Revolute Idler F/RConn2 -- PS-SL IdlerF/LConn1
